simulink model "Z3"  (R2015b)
settings: Solver=VariableStepAuto  StartTime=0.0  StopTime=20.0  RelTol=1e-3
settings Model: Creator=Erdal  LastModifiedBy=Erdal

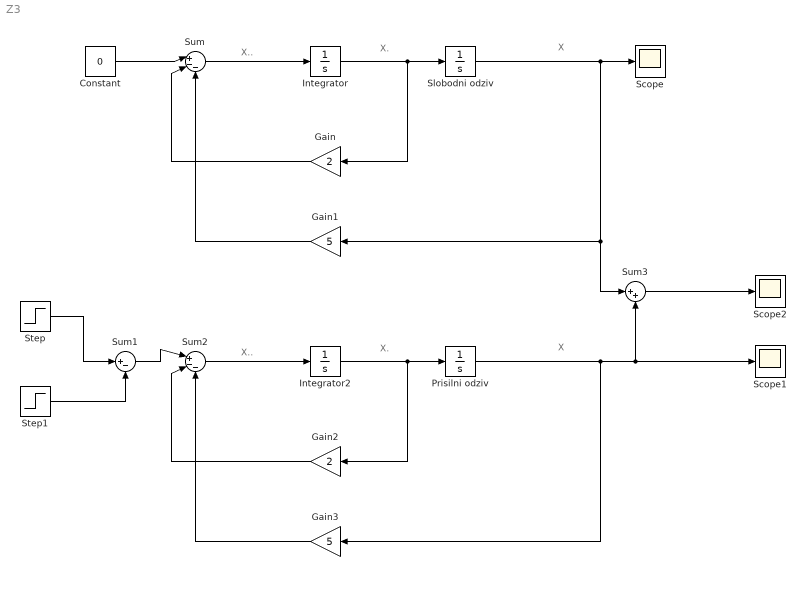
== system Z3 ==
  note: X
  note: X.
  note: X..
  note: X
  note: X.
  note: X..
  Constant : Constant  Value=0
  Gain : Gain  Gain=2
  Gain1 : Gain  Gain=5
  Gain2 : Gain  Gain=2
  Gain3 : Gain  Gain=5
  Integrator : Integrator  InitialCondition=1
  Integrator2 : Integrator
  Prisilni odziv : Integrator
  Scope : Scope
  Scope1 : Scope
  Scope2 : Scope
  Slobodni odziv : Integrator  InitialCondition=1
  Step : Step  Time=5  SampleTime=0
  Step1 : Step  Time=10  SampleTime=0
  Sum : Sum  Inputs=|+--
  Sum1 : Sum  Inputs=|+-
  Sum2 : Sum  Inputs=|+--
  Sum3 : Sum  Inputs=|++
  wires:
  Step/1 -> Sum1/1
  Step1/1 -> Sum1/2
  Constant/1 -> Sum/1
  Sum/1 -> Integrator/1
  Integrator/1 -> Gain/1, Slobodni odziv/1
  Slobodni odziv/1 -> Sum3/1, Gain1/1, Scope/1
  Gain/1 -> Sum/2
  Gain1/1 -> Sum/3
  Sum2/1 -> Integrator2/1
  Integrator2/1 -> Prisilni odziv/1, Gain2/1
  Prisilni odziv/1 -> Sum3/2, Scope1/1, Gain3/1
  Gain2/1 -> Sum2/2
  Gain3/1 -> Sum2/3
  Sum1/1 -> Sum2/1
  Sum3/1 -> Scope2/1
